simulink subsystem "PackActorPose"  (R2024b)
settings: Solver=VariableStepAuto  StartTime=0.0  StopTime=10.0  RelTol=1e-3
undefined symbols (not defined in the file or in its folder): ActorID, AngularVelocity, DiscIntNeverNeededParam, Pose, Velocity
settings Model: Creator=The MathWorks, Inc.  LastModifiedBy=The MathWorks, Inc.
settings OptimizationCC: ReuseModelBlockBuffer=off
settings RTWCC: GPUComputeCapability=3.5

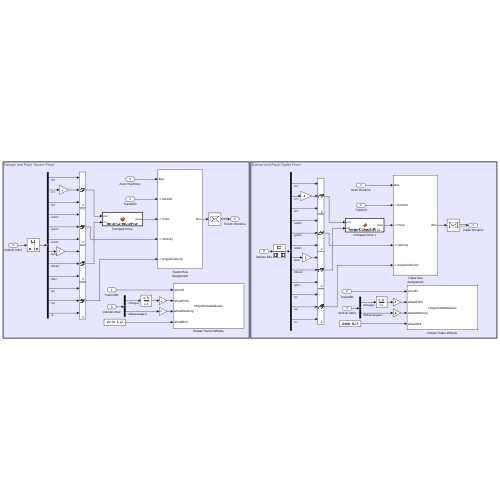
[thumbnail: Simulink's stored preview of the top-level diagram]
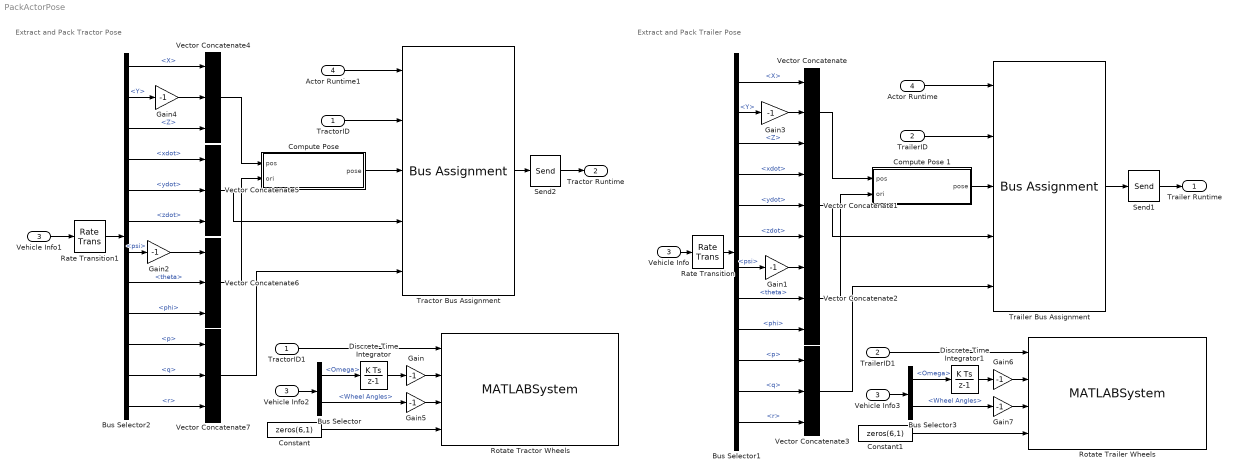
== system PackActorPose ==
  note: Extract and Pack Tractor Pose
  note: Extract and Pack Trailer Pose
  TractorID : Inport
  TrailerID : Inport  Port=2
  Vehicle Info : Inport  Port=3
  Actor Runtime : Inport  Port=4
  Actor Runtime1 : InportShadow  Port=4
  Bus Selector : BusSelector  OutputSignals=Tractor.Wheels.TireFrame.Omega,Tractor.Wheels.Steering.Wheel Angles
  Bus Selector1 : BusSelector  OutputSignals=Trailer.Vehicle.InertFrm.Geom.Disp.X,Trailer.Vehicle.InertFrm.Geom.Disp.Y,Trailer.Vehicle.InertFrm.Cg.Disp.Z,Trailer.Vehicle.BdyFrm.Cg.Vel.xdot,Trailer.Vehicle.BdyFrm.Cg.Vel.ydot,Trailer.Vehicle.BdyFrm.Cg.Vel.zdot,Trailer.Vehicle.InertFrm.Cg.Ang.psi,Trailer.Vehicle.InertFrm.Cg.Ang.theta,Trailer.Vehicle.InertFrm.Cg.Ang.phi,Trailer.Vehicle.BdyFrm.Cg.AngVel.p,Trailer.Vehicle.BdyFrm.Cg.AngVel.q,Trailer.Vehicle.BdyFrm.Cg.AngVel.r
  Bus Selector2 : BusSelector  OutputSignals=Tractor.Vehicle.InertFrm.Geom.Disp.X,Tractor.Vehicle.InertFrm.Geom.Disp.Y,Tractor.Vehicle.InertFrm.Cg.Disp.Z,Tractor.Vehicle.BdyFrm.Cg.Vel.xdot,Tractor.Vehicle.BdyFrm.Cg.Vel.ydot,Tractor.Vehicle.BdyFrm.Cg.Vel.zdot,Tractor.Vehicle.InertFrm.Cg.Ang.psi,Tractor.Vehicle.InertFrm.Cg.Ang.theta,Tractor.Vehicle.InertFrm.Cg.Ang.phi,Tractor.Vehicle.BdyFrm.Cg.AngVel.p,Tractor.Vehicle.BdyFrm.Cg.AngVel.q,Tractor.Vehicle.BdyFrm.Cg.AngVel.r
  Bus Selector3 : BusSelector  OutputSignals=Trailer.Wheels.TireFrame.Omega,Trailer.Wheels.Steering.Wheel Angles
  Compute Pose : MATLAB Function  TreatAsAtomicUnit=on
  Compute Pose 1 : MATLAB Function  TreatAsAtomicUnit=on
  Constant : Constant  Value=zeros(6,1)
  Constant1 : Constant  Value=zeros(6,1)
  Discrete-Time Integrator : DiscreteIntegrator  SampleTime=-1  ICPrevOutput=DiscIntNeverNeededParam  ICPrevScaledInput=DiscIntNeverNeededParam
  Discrete-Time Integrator1 : DiscreteIntegrator  SampleTime=-1  ICPrevOutput=DiscIntNeverNeededParam  ICPrevScaledInput=DiscIntNeverNeededParam
  Gain{,1..7} (8 alike) : Gain  Gain=-1
  Rate Transition : RateTransition  OutPortSampleTime=Ts
  Rate Transition1 : RateTransition  OutPortSampleTime=Ts
  Rotate Tractor Wheels : MATLABSystem  System=HelperRotateWheels
      mask Type: HelperRotateWheels
      mask Display:
      | disp('HelperRotateWheels');
      | port_label('input',1,'actorID');
      | port_label('input',2,'wheelPitch');
      | port_label('input',3,'wheelSteering');
      | port_label('input',4,'wheelRoll');
  Rotate Trailer Wheels : MATLABSystem  System=HelperRotateWheels
      mask Type: HelperRotateWheels
      mask Display:
      | disp('HelperRotateWheels');
      | port_label('input',1,'actorID');
      | port_label('input',2,'wheelPitch');
      | port_label('input',3,'wheelSteering');
      | port_label('input',4,'wheelRoll');
  Send1 : Send  OutputPortMessageModes=m
  Send2 : Send  OutputPortMessageModes=m
  Tractor Bus Assignment : BusAssignment  AssignedSignals=ActorID,Pose,Velocity,AngularVelocity
  TractorID1 : InportShadow
  Trailer Bus Assignment : BusAssignment  AssignedSignals=ActorID,Pose,Velocity,AngularVelocity
  TrailerID1 : InportShadow  Port=2
  Vector Concatenate{,1..7} (8 alike) : Concatenate  NumInputs=3  Mode=Multidimensional array  ConcatenateDimension=2
  Vehicle Info1 : InportShadow  Port=3
  Vehicle Info2 : InportShadow  Port=3
  Vehicle Info3 : InportShadow  Port=3
  Trailer Runtime : Outport
  Tractor Runtime : Outport  Port=2
  wires:
  Trailer Bus Assignment/1 -> Send1/1
  Send1/1 -> Trailer Runtime/1
  Bus Selector1/9 -> Vector Concatenate2/3  "<phi>"
  Gain1/1 -> Vector Concatenate2/1
  Gain3/1 -> Vector Concatenate/2
  Bus Selector1/12 -> Vector Concatenate3/3  "<r>"
  Bus Selector1/11 -> Vector Concatenate3/2  "<q>"
  Bus Selector1/10 -> Vector Concatenate3/1  "<p>"
  Bus Selector1/8 -> Vector Concatenate2/2  "<theta>"
  Bus Selector1/7 -> Gain1/1  "<psi>"
  Bus Selector1/6 -> Vector Concatenate1/3  "<zdot>"
  Bus Selector1/5 -> Vector Concatenate1/2  "<ydot>"
  Bus Selector1/4 -> Vector Concatenate1/1  "<xdot>"
  Bus Selector1/3 -> Vector Concatenate/3  "<Z>"
  Bus Selector1/2 -> Gain3/1  "<Y>"
  Bus Selector1/1 -> Vector Concatenate/1  "<X>"
  Compute Pose 1/1(pose) -> Trailer Bus Assignment/3
  TrailerID/1 -> Trailer Bus Assignment/2
  Vector Concatenate/1 -> Compute Pose 1/1(pos)
  Bus Selector2/9 -> Vector Concatenate6/3  "<phi>"
  Gain2/1 -> Vector Concatenate6/1
  Bus Selector2/3 -> Vector Concatenate4/3  "<Z>"
  Bus Selector2/7 -> Gain2/1  "<psi>"
  Bus Selector2/10 -> Vector Concatenate7/1  "<p>"
  Gain4/1 -> Vector Concatenate4/2
  Bus Selector2/1 -> Vector Concatenate4/1  "<X>"
  Bus Selector2/8 -> Vector Concatenate6/2  "<theta>"
  Bus Selector2/4 -> Vector Concatenate5/1  "<xdot>"
  Bus Selector2/5 -> Vector Concatenate5/2  "<ydot>"
  Bus Selector2/6 -> Vector Concatenate5/3  "<zdot>"
  Bus Selector2/12 -> Vector Concatenate7/3  "<r>"
  Bus Selector2/11 -> Vector Concatenate7/2  "<q>"
  Bus Selector2/2 -> Gain4/1  "<Y>"
  Vehicle Info1/1 -> Rate Transition1/1
  Vehicle Info/1 -> Rate Transition/1
  Rate Transition/1 -> Bus Selector1/1
  Rate Transition1/1 -> Bus Selector2/1
  Actor Runtime/1 -> Trailer Bus Assignment/1
  Vector Concatenate2/1 -> Compute Pose 1/2(ori)
  Send2/1 -> Tractor Runtime/1
  Vector Concatenate6/1 -> Compute Pose/2(ori)
  TractorID/1 -> Tractor Bus Assignment/2
  Tractor Bus Assignment/1 -> Send2/1
  Vector Concatenate4/1 -> Compute Pose/1(pos)
  Vector Concatenate7/1 -> Tractor Bus Assignment/5
  Vector Concatenate1/1 -> Trailer Bus Assignment/4
  Vector Concatenate3/1 -> Trailer Bus Assignment/5
  Compute Pose/1(pose) -> Tractor Bus Assignment/3
  Vector Concatenate5/1 -> Tractor Bus Assignment/4
  Actor Runtime1/1 -> Tractor Bus Assignment/1
  TractorID1/1 -> Rotate Tractor Wheels/1
  Vehicle Info2/1 -> Bus Selector/1
  Bus Selector/2 -> Gain5/1  "<Wheel Angles>"
  Bus Selector/1 -> Discrete-Time Integrator/1  "<Omega>"
  Constant/1 -> Rotate Tractor Wheels/4
  Discrete-Time Integrator/1 -> Gain/1
  Vehicle Info3/1 -> Bus Selector3/1
  TrailerID1/1 -> Rotate Trailer Wheels/1
  Discrete-Time Integrator1/1 -> Gain6/1
  Constant1/1 -> Rotate Trailer Wheels/4
  Bus Selector3/1 -> Discrete-Time Integrator1/1  "<Omega>"
  Bus Selector3/2 -> Gain7/1  "<Wheel Angles>"
  Gain/1 -> Rotate Tractor Wheels/2
  Gain5/1 -> Rotate Tractor Wheels/3
  Gain6/1 -> Rotate Trailer Wheels/2
  Gain7/1 -> Rotate Trailer Wheels/3

== matlab function PackActorPose/Compute Pose 1 ==
  data: pos input; pose output; ori input
function pose = helperComputePose(pos,ori)
    rotm = zeros(3,3);
    pose = zeros(4,4);
    rotm = eul2rotm([-pi/2 0 0]+ori);
    pose = [[rotm pos']; [0 0 0 1]];
end

== matlab function PackActorPose/Compute Pose ==
  data: pos input; pose output; ori input
function pose = helperComputePose(pos,ori)
    rotm = zeros(3,3);
    pose = zeros(4,4);
    rotm = eul2rotm([-pi/2 0 0]+ori);
    pose = [[rotm pos']; [0 0 0 1]];
end
